simulink library "udp_powerfactor_lib"  (Simulink 8.1)
settings: Solver=ode45  StartTime=0.0  StopTime=10.0  RelTol=1e-3
undefined symbols (not defined in the file): Ts
libraries: simulink x7, powerlib_extras x2
settings Model: Creator=re25624  LastModifiedBy=re25624

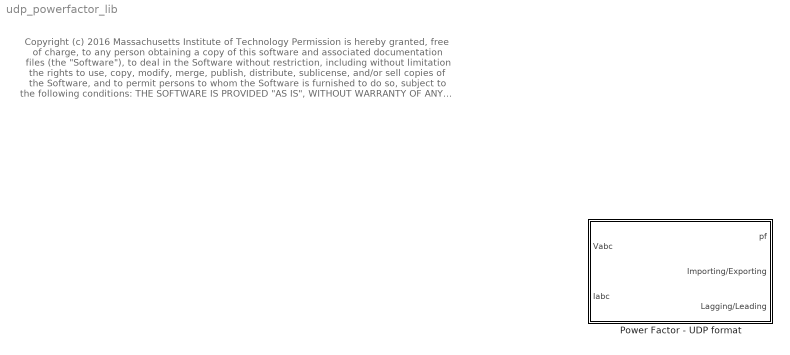
== system udp_powerfactor_lib ==
  note: Copyright (c) 2016 Massachusetts Institute of Technology
      | Permission is hereby granted, free of charge, to any person obtaining a copy of this software and associated documentation files (the "Software"), to deal
      | in the Software without restriction, including without limitation the rights to use, copy, modify, merge, publish, distribute, sublicense, and/or sell copies of the
      | Software, and to permit persons to whom the Software is furnished to do so, subject to the following conditions:
      |
      | THE SOFTWARE IS PROVIDED "AS IS", WITHOUT WARRANTY OF ANY KIND, EXPRESS OR IMPLIED, INCLUDING BUT NOT LIMITED TO THE
      | WARRANTIES OF MERCHANTABILITY, FITNESS FOR A PARTICULAR PURPOSE AND NONINFRINGEMENT. IN NO EVENT SHALL THE AUTHORS
      | OR COPYRIGHT HOLDERS BE LIABLE FOR ANY CLAIM, DAMAGES OR OTHER LIABILITY, WHETHER IN AN ACTION OF CONTRACT, TORT OR
      | OTHERWISE, ARISING FROM, OUT OF OR IN CONNECTION WITH THE SOFTWARE OR THE USE OR OTHER DEALINGS IN THE SOFTWARE
  Power Factor - UDP format : Subsystem

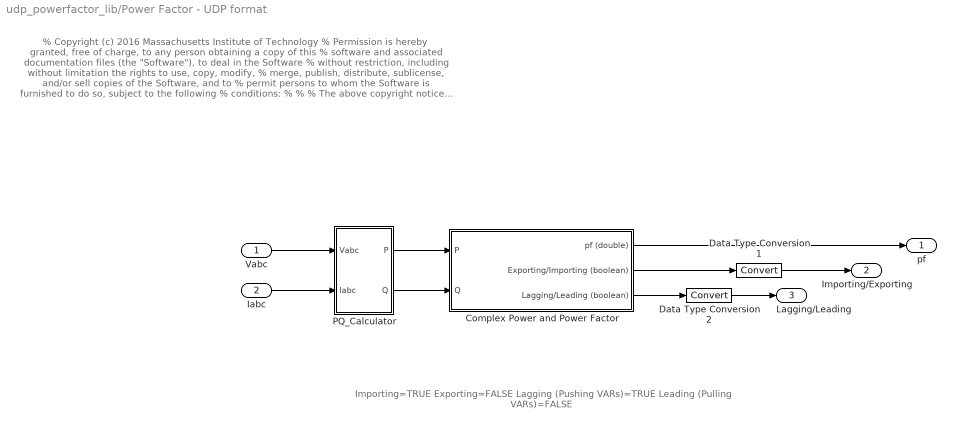
== system udp_powerfactor_lib/Power Factor - UDP format ==
  note: % Copyright (c) 2016 Massachusetts Institute of Technology
      | % Permission is hereby granted, free of charge, to any person obtaining a copy of this
      | % software and associated documentation files (the "Software"), to deal in the Software
      | % without restriction, including without limitation the rights to use, copy, modify,
      | % merge, publish, distribute, sublicense, and/or sell copies of the Software, and to
      | % permit persons to whom the Software is furnished to do so, subject to the following
      | % conditions:
      | %
      | %
      | % The above copyright notice and this permission notice shall be included in
      | % all copies or substantial portions of the Software.
      | %
      | % THE SOFTWARE IS PROVIDED "AS IS", WITHOUT WARRANTY OF ANY KIND, EXPRESS OR IMPLIED,
      | % INCLUDING BUT NOT LIMITED TO THE WARRANTIES OF MERCHANTABILITY, FITNESS FOR A
      | % PARTICULAR PURPOSE AND NONINFRINGEMENT. IN NO EVENT SHALL THE AUTHORS OR COPYRIGHT
      | % HOLDERS BE LIABLE FOR ANY CLAIM, DAMAGES OR OTHER LIABILITY, WHETHER IN AN ACTION
      | % OF CONTRACT, TORT OR OTHERWISE, ARISING FROM, OUT OF OR IN CONNECTION WITH THE
      | % SOFTWARE OR THE USE OR OTHER DEALINGS IN THE SOFTWARE.
      | %
      | %
      | %%
  note: Importing=TRUE
      | Exporting=FALSE
      |
      | Lagging (Pushing VARs)=TRUE
      | Leading (Pulling VARs)=FALSE
  Vabc : Inport
  Iabc : Inport  Port=2
  Complex Power and Power Factor : Subsystem
  Data Type Conversion1 : DataTypeConversion
  Data Type Conversion2 : DataTypeConversion
  PQ_Calculator : Subsystem
  pf : Outport
  Importing/Exporting : Outport  Port=2
  Lagging/Leading : Outport  Port=3
  wires:
  Data Type Conversion1/1 -> Importing/Exporting/1
  Data Type Conversion2/1 -> Lagging/Leading/1
  Complex Power and Power Factor/2(Exporting/Importing (boolean)) -> Data Type Conversion1/1
  Complex Power and Power Factor/3(Lagging/Leading (boolean)) -> Data Type Conversion2/1
  PQ_Calculator/1(P) -> Complex Power and Power Factor/1(P)
  PQ_Calculator/2(Q) -> Complex Power and Power Factor/2(Q)
  Complex Power and Power Factor/1(pf (double)) -> pf/1
  Vabc/1 -> PQ_Calculator/1(Vabc)
  Iabc/1 -> PQ_Calculator/2(Iabc)

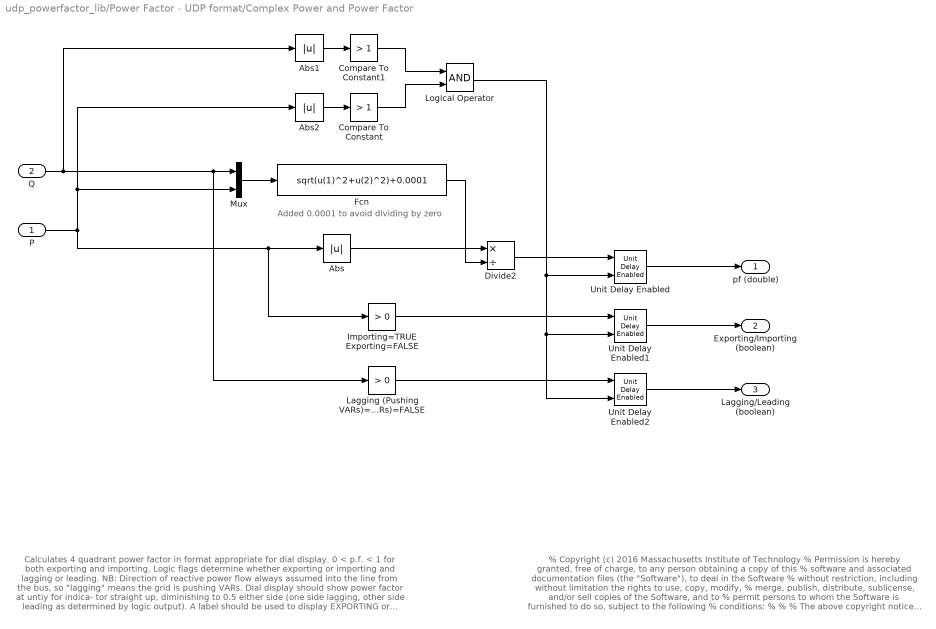
== system udp_powerfactor_lib/Power Factor - UDP format/Complex Power and Power Factor ==
  note: % Copyright (c) 2016 Massachusetts Institute of Technology
      | % Permission is hereby granted, free of charge, to any person obtaining a copy of this
      | % software and associated documentation files (the "Software"), to deal in the Software
      | % without restriction, including without limitation the rights to use, copy, modify,
      | % merge, publish, distribute, sublicense, and/or sell copies of the Software, and to
      | % permit persons to whom the Software is furnished to do so, subject to the following
      | % conditions:
      | %
      | %
      | % The above copyright notice and this permission notice shall be included in
      | % all copies or substantial portions of the Software.
      | %
      | % THE SOFTWARE IS PROVIDED "AS IS", WITHOUT WARRANTY OF ANY KIND, EXPRESS OR IMPLIED,
      | % INCLUDING BUT NOT LIMITED TO THE WARRANTIES OF MERCHANTABILITY, FITNESS FOR A
      | % PARTICULAR PURPOSE AND NONINFRINGEMENT. IN NO EVENT SHALL THE AUTHORS OR COPYRIGHT
      | % HOLDERS BE LIABLE FOR ANY CLAIM, DAMAGES OR OTHER LIABILITY, WHETHER IN AN ACTION
      | % OF CONTRACT, TORT OR OTHERWISE, ARISING FROM, OUT OF OR IN CONNECTION WITH THE
      | % SOFTWARE OR THE USE OR OTHER DEALINGS IN THE SOFTWARE.
      | %
      | %
      | %%
  note: Calculates 4 quadrant power factor in format appropriate
      | for dial display.  0 < p.f. < 1 for both exporting and
      | importing.  Logic flags determine whether exporting or
      | importing and lagging or leading.  NB:  Direction of
      | reactive power flow always assumed into the line from the
      | bus, so "lagging" means the grid is pushing VARs.
      |
      | Dial display should show power factor at untiy for indica-
      | tor straight up, diminishing to 0.5 either side (one side
      | lagging, other side leading as determined by logic output).
      | A label should be used to display EXPORTING or IMPORTING
      | based on logic output.
  note: Added 0.0001 to avoid dividing by zero
  P : Inport
  Q : Inport  Port=2
  Abs : Abs
  Abs1 : Abs
  Abs2 : Abs
  Compare To Constant : simulink/Logic and Bit Operations/Compare To Constant  relop=>  const=1  OutDataTypeStr=uint8
  Compare To Constant1 : simulink/Logic and Bit Operations/Compare To Constant  relop=>  const=1  OutDataTypeStr=uint8
  Divide2 : Product  Inputs=*/
  Fcn : Fcn  Expr=sqrt(u(1)^2+u(2)^2)+0.0001
  Importing=TRUE Exporting=FALSE : simulink/Logic and Bit Operations/Compare To Constant  relop=>  const=0  OutDataTypeStr=boolean
  Lagging (Pushing VARs)=TRUE Leading (Pulling VARs)=FALSE : simulink/Logic and Bit Operations/Compare To Constant  relop=>  const=0  OutDataTypeStr=boolean
  Logical Operator : Logic  AllPortsSameDT=off  OutDataTypeStr=boolean
  Mux : Mux  Inputs=2
  Unit Delay Enabled : simulink/Additional Math & Discrete/Additional Discrete/Unit Delay Enabled  vinit=1  tsamp=-1
  Unit Delay Enabled1 : simulink/Additional Math & Discrete/Additional Discrete/Unit Delay Enabled  vinit=1  tsamp=-1
  Unit Delay Enabled2 : simulink/Additional Math & Discrete/Additional Discrete/Unit Delay Enabled  vinit=1  tsamp=-1
  pf (double) : Outport
  Exporting/Importing (boolean) : Outport  Port=2
  Lagging/Leading (boolean) : Outport  Port=3
  wires:
  Fcn/1 -> Divide2/2
  P/1 -> Abs/1, Importing=TRUE Exporting=FALSE/1, Mux/2, Abs2/1
  Q/1 -> Mux/1, Lagging (Pushing VARs)=TRUE Leading (Pulling VARs)=FALSE/1, Abs1/1
  Mux/1 -> Fcn/1
  Abs/1 -> Divide2/1
  Divide2/1 -> Unit Delay Enabled/1
  Unit Delay Enabled/1 -> pf (double)/1
  Importing=TRUE Exporting=FALSE/1 -> Unit Delay Enabled1/1
  Unit Delay Enabled1/1 -> Exporting/Importing (boolean)/1
  Lagging (Pushing VARs)=TRUE Leading (Pulling VARs)=FALSE/1 -> Unit Delay Enabled2/1
  Unit Delay Enabled2/1 -> Lagging/Leading (boolean)/1
  Abs2/1 -> Compare To Constant/1
  Abs1/1 -> Compare To Constant1/1
  Compare To Constant1/1 -> Logical Operator/1
  Compare To Constant/1 -> Logical Operator/2
  Logical Operator/1 -> Unit Delay Enabled/2, Unit Delay Enabled1/2, Unit Delay Enabled2/2

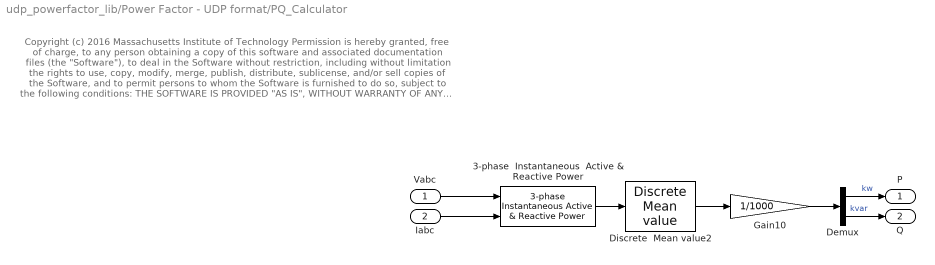
== system udp_powerfactor_lib/Power Factor - UDP format/PQ_Calculator ==
  note: Copyright (c) 2016 Massachusetts Institute of Technology
      | Permission is hereby granted, free of charge, to any person obtaining a copy of this software and associated documentation files (the "Software"), to deal
      | in the Software without restriction, including without limitation the rights to use, copy, modify, merge, publish, distribute, sublicense, and/or sell copies of the
      | Software, and to permit persons to whom the Software is furnished to do so, subject to the following conditions:
      |
      | THE SOFTWARE IS PROVIDED "AS IS", WITHOUT WARRANTY OF ANY KIND, EXPRESS OR IMPLIED, INCLUDING BUT NOT LIMITED TO THE
      | WARRANTIES OF MERCHANTABILITY, FITNESS FOR A PARTICULAR PURPOSE AND NONINFRINGEMENT. IN NO EVENT SHALL THE AUTHORS
      | OR COPYRIGHT HOLDERS BE LIABLE FOR ANY CLAIM, DAMAGES OR OTHER LIABILITY, WHETHER IN AN ACTION OF CONTRACT, TORT OR
      | OTHERWISE, ARISING FROM, OUT OF OR IN CONNECTION WITH THE SOFTWARE OR THE USE OR OTHER DEALINGS IN THE SOFTWARE
  Vabc : Inport
  Iabc : Inport  Port=2
  3-phase  Instantaneous  Active & Reactive Power : powerlib_extras/Measurements/3-phase  Instantaneous  Active & Reactive Power
  Demux : Demux  Outputs=2
  Discrete  Mean value2 : powerlib_extras/Discrete Measurements/Discrete  Mean value  Freq=60  Vinit=0  Ts=Ts
  Gain10 : Gain  Gain=1/1000
  P : Outport
  Q : Outport  Port=2
  wires:
  Demux/2 -> Q/1  "kvar"
  Demux/1 -> P/1  "kw"
  Iabc/1 -> 3-phase  Instantaneous  Active & Reactive Power/2
  Vabc/1 -> 3-phase  Instantaneous  Active & Reactive Power/1
  Discrete  Mean value2/1 -> Gain10/1
  3-phase  Instantaneous  Active & Reactive Power/1 -> Discrete  Mean value2/1
  Gain10/1 -> Demux/1
